simulink model "model_5LinkWalking_NODS"  (R2022b)
settings: Solver=VariableStepAuto  StartTime=0.0  StopTime=Tf  FixedStep=1e-5  MaxStep=1e-3  RelTol=1e-12  AbsTol=1e-8
values from neighbouring files (symbols this model uses):
  dq0 = [ocl_traj.simout(N,6); ocl_traj.simout(N,7); ocl_traj.simout(N,8); ocl_traj.simout(N,9); ocl_traj.simout(N,10)]    [run_walking_simulation.m]    (also in run_walking_simulation_parallel.m; search_delta_bar_parallel.m)
  gains = [K_p,K_d,K_p,K_d,K_p,K_d,K_p,K_d,K_p,K_d]    [main.m]
  init_flag = [-1; 0; ocl_traj.x_sw(1); init_t_mode_change; alpha_ref(1); 0; y_g_curr]    [run_walking_simulation.m]
  Initial_state = [q0;dq0]    [run_walking_simulation.m]    (also in run_walking_simulation_parallel.m; search_delta_bar_parallel.m)
  inputs_ref = [step_alpha_ref, step_inputs_ref]    [run_walking_simulation.m]
  joint_angles_ref = [ocl_traj.time, ocl_traj.simout, alpha_ref]    [run_walking_simulation.m]    (also in run_walking_simulation_parallel.m; search_delta_bar_parallel.m)
  landing_ref = [landing_traj.time, landing_traj.simout, alpha_ref_landing]    [run_walking_simulation.m]    (also in run_walking_simulation_parallel.m; search_delta_bar_parallel.m)
  param = [params.m1; params.m2; params.m5; params.l1; params.l2; params.l5; params.g; params.I1; params.I2; params.I5; params.r_k; params.r_h; params.k_ba; params.phi_h0; params.phi_k0]    [main.m]    (also in run_walking_simulation.m; run_walking_simulation_parallel.m)
  q0 = [ocl_traj.simout(N,1); ocl_traj.simout(N,2); ocl_traj.simout(N,3); ocl_traj.simout(N,4); ocl_traj.simout(N,5)]    [run_walking_simulation.m]    (also in run_walking_simulation_parallel.m; search_delta_bar_parallel.m)
  sample_time = 0.001    [run_walking_simulation.m]    (also in run_walking_simulation_parallel.m; search_delta_bar_parallel.m)
undefined symbols (not defined in the file or in its folder): uneven_terrain
libraries: simulink x2
(part 1 of 2)
settings Model: SimulationMode=accelerator  Creator=yamakita_lab  LastModifiedBy=mmpel
settings SolverCC: AutoScaleAbsTol=off  AlgebraicLoopSolver=TrustRegion
settings DataIOCC: ReturnWorkspaceOutputs=off
settings DebuggingCC: ParameterPrecisionLossMsg=none  UnconnectedInputMsg=warning  UnconnectedOutputMsg=warning  UnconnectedLineMsg=warning  SFMachineParentedDataDiag=warning  ArithmeticOperatorsInVariantConditions=warning
settings ModelReferenceCC: EnableRefExpFcnMdlSchedulingChecks=on
settings SFSimCC: SimUseLocalCustomCode=off  CustomCodeUndefinedFunction=UseInterfaceOnly
settings RTWCC: RTWUseLocalCustomCode=off  DLArmComputeVersion=19.05

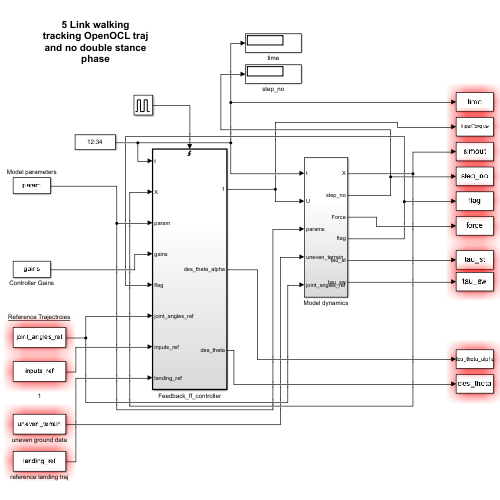
[thumbnail: Simulink's stored preview of the top-level diagram]
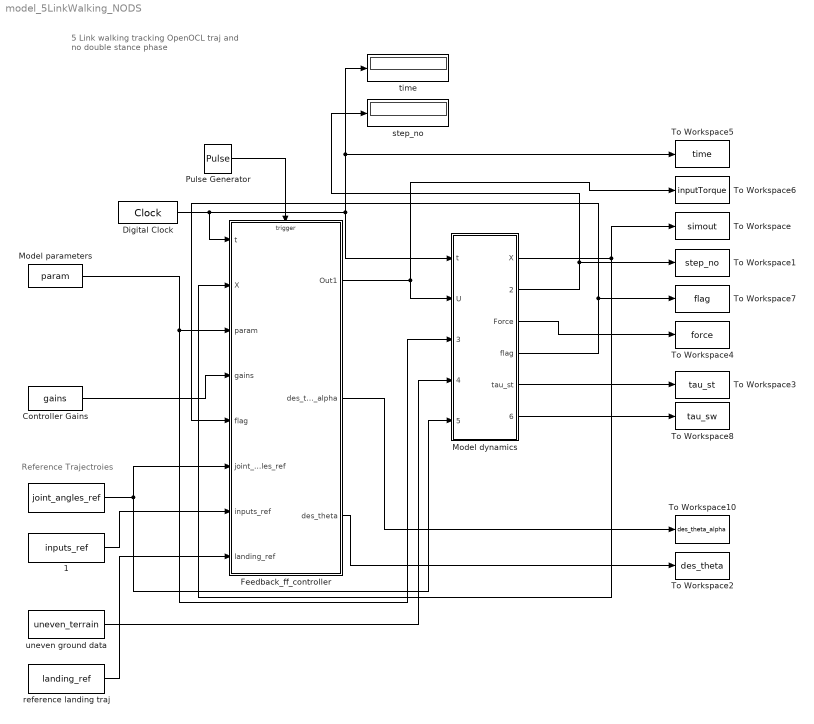
== system model_5LinkWalking_NODS ==
  note: Reference Trajectroies
  note: 5 Link walking tracking OpenOCL traj and no double stance phase
  " " : Constant  Value=joint_angles_ref
  " 1" : Constant  Value=inputs_ref
  Controller Gains : Constant  Value=gains
  Digital Clock : DigitalClock  SampleTime=1e-4
  Feedback_ff_controller : Subsystem  TreatAsAtomicUnit=on
  Model dynamics : Subsystem
  Model parameters : Constant  Value=param  OutDataTypeStr=double
  Pulse Generator : DiscretePulseGenerator  PulseType=Time based  Period=5e-4  PulseWidth=5
  To Workspace : ToWorkspace  VariableName=simout  SampleTime=sample_time
  To Workspace1 : ToWorkspace  VariableName=step_no  SampleTime=sample_time
  To Workspace10 : ToWorkspace  VariableName=des_theta_alpha  SampleTime=sample_time
  To Workspace2 : ToWorkspace  VariableName=des_theta  SampleTime=sample_time
  To Workspace3 : ToWorkspace  VariableName=tau_st  SampleTime=sample_time
  To Workspace4 : ToWorkspace  VariableName=force  SampleTime=sample_time
  To Workspace5 : ToWorkspace  VariableName=time  SampleTime=sample_time
  To Workspace6 : ToWorkspace  VariableName=inputTorque  SampleTime=sample_time
  To Workspace7 : ToWorkspace  VariableName=flag  SampleTime=sample_time
  To Workspace8 : ToWorkspace  VariableName=tau_sw  SampleTime=sample_time
  reference landing traj : Constant  Value=landing_ref
  step_no : Display
  time : Display
  uneven ground data : Constant  Value=uneven_terrain  OutDataTypeStr=Bus: uneven_terrain_bus
  wires:
  Feedback_ff_controller/1(Out1) -> Model dynamics/2(U), To Workspace6/1
  Model dynamics/1(X) -> To Workspace/1, Feedback_ff_controller/2(X)
  Digital Clock/1 -> time/1, To Workspace5/1, Model dynamics/1(t), Feedback_ff_controller/1(t)
  Model dynamics/2(step_no) -> step_no/1, To Workspace1/1
  Model dynamics/3(Force) -> To Workspace4/1
  Model parameters/1 -> Model dynamics/3(params), Feedback_ff_controller/3(param)
  Controller Gains/1 -> Feedback_ff_controller/4(gains)
  Model dynamics/4(flag) -> To Workspace7/1, Feedback_ff_controller/5(flag)
  " "/1 -> Model dynamics/5(joint_angles_ref), Feedback_ff_controller/6(joint_angles_ref)
  Pulse Generator/1 -> Feedback_ff_controller/Trigger
  Model dynamics/5(tau_st) -> To Workspace3/1
  Model dynamics/6(tau_sw) -> To Workspace8/1
  " 1"/1 -> Feedback_ff_controller/7(inputs_ref)
  Feedback_ff_controller/2(des_theta_alpha) -> To Workspace10/1
  Feedback_ff_controller/3(des_theta) -> To Workspace2/1
  uneven ground data/1 -> Model dynamics/4(uneven_terrain)
  reference landing traj/1 -> Feedback_ff_controller/8(landing_ref)

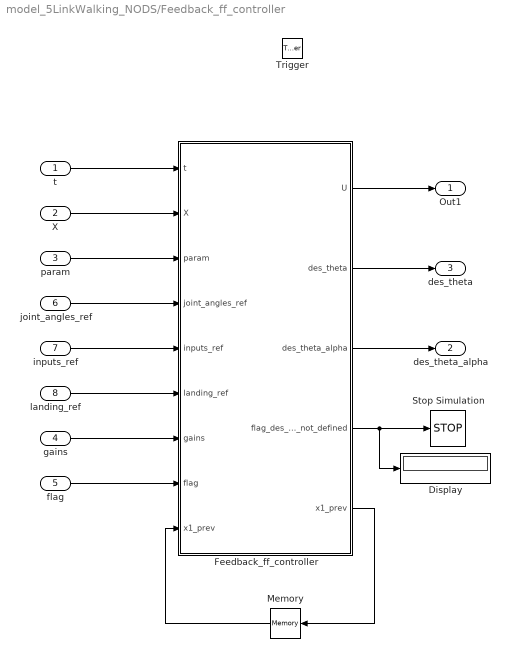
== system model_5LinkWalking_NODS/Feedback_ff_controller ==
  t : Inport
  X : Inport  Port=2
  param : Inport  Port=3
  gains : Inport  Port=4
  flag : Inport  Port=5
  joint_angles_ref : Inport  Port=6
  inputs_ref : Inport  Port=7
  landing_ref : Inport  Port=8
  Trigger : TriggerPort  VariantControl=Variant  PortDimensions=1
  Display : Display
  Feedback_ff_controller : MATLAB Function  TreatAsAtomicUnit=on
  Memory : Memory  InitialCondition=[0, 0]  InheritSampleTime=on
  Stop Simulation : Stop
  Out1 : Outport  VectorParamsAs1DForOutWhenUnconnected=off
  des_theta_alpha : Outport  Port=2  InitialOutput=[q0; dq0; 0]  VectorParamsAs1DForOutWhenUnconnected=off
  des_theta : Outport  Port=3  InitialOutput=[q0; dq0]  VectorParamsAs1DForOutWhenUnconnected=off
  wires:
  Feedback_ff_controller/1(U) -> Out1/1
  t/1 -> Feedback_ff_controller/1(t)
  X/1 -> Feedback_ff_controller/2(X)
  param/1 -> Feedback_ff_controller/3(param)
  Memory/1 -> Feedback_ff_controller/9("x1_prev ")
  Feedback_ff_controller/5(x1_prev) -> Memory/1
  gains/1 -> Feedback_ff_controller/7(gains)
  flag/1 -> Feedback_ff_controller/8(flag)
  joint_angles_ref/1 -> Feedback_ff_controller/4(joint_angles_ref)
  inputs_ref/1 -> Feedback_ff_controller/5(inputs_ref)
  Feedback_ff_controller/3(des_theta_alpha) -> des_theta_alpha/1
  Feedback_ff_controller/2(des_theta) -> des_theta/1
  landing_ref/1 -> Feedback_ff_controller/6(landing_ref)
  Feedback_ff_controller/4(flag_des_theta_not_defined) -> Display/1, Stop Simulation/1

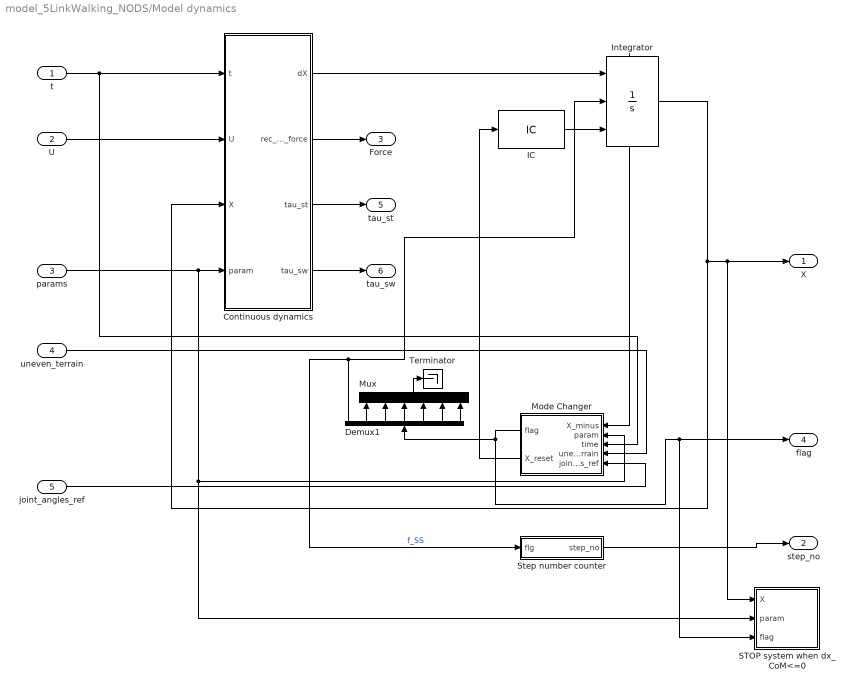
== system model_5LinkWalking_NODS/Model dynamics ==
  t : Inport
  U : Inport  Port=2
  params : Inport  Port=3
  uneven_terrain : Inport  Port=4
  joint_angles_ref : Inport  Port=5
  Continuous dynamics : MATLAB Function  TreatAsAtomicUnit=on
  Demux1 : Demux  Outputs=7
  IC : InitialCondition  Value=Initial_state
  Integrator : Integrator  ExternalReset=rising  InitialConditionSource=external  ShowStatePort=on
  Mode Changer : Subsystem
  Mux : Mux  Inputs=6
  STOP system when dx_CoM<=0 : Subsystem
  Step number counter : Subsystem
  Terminator : Terminator
  X : Outport  VectorParamsAs1DForOutWhenUnconnected=off
  step_no : Outport  Port=2  VectorParamsAs1DForOutWhenUnconnected=off
  Force : Outport  Port=3  VectorParamsAs1DForOutWhenUnconnected=off
  flag : Outport  Port=4
  tau_st : Outport  Port=5  VectorParamsAs1DForOutWhenUnconnected=off
  tau_sw : Outport  Port=6  VectorParamsAs1DForOutWhenUnconnected=off
  wires:
  IC/1 -> Integrator/3
  Integrator/State -> Mode Changer/1(X_minus)
  Continuous dynamics/1(dX) -> Integrator/1
  params/1 -> Continuous dynamics/4(param), STOP system when dx_CoM<=0/2(param), Mode Changer/2("param ")
  U/1 -> Continuous dynamics/2(U)
  t/1 -> Continuous dynamics/1(t), Mode Changer/3(time)
  Integrator/1 -> STOP system when dx_CoM<=0/1(X), X/1, Continuous dynamics/3(X)
  Mode Changer/2(X_reset) -> IC/1
  Mode Changer/1(flag) -> STOP system when dx_CoM<=0/3(flag), flag/1, Demux1/1
  Demux1/1 -> Integrator/2, Step number counter/1(flg)  "f_SS"
  Step number counter/1(step_no) -> step_no/1
  Continuous dynamics/2(rec_cs_force) -> Force/1
  Continuous dynamics/3(tau_st) -> tau_st/1
  Continuous dynamics/4(tau_sw) -> tau_sw/1
  Demux1/2 -> Mux/1
  Demux1/3 -> Mux/2
  Demux1/4 -> Mux/3
  Demux1/5 -> Mux/4
  Demux1/6 -> Mux/5
  Mux/1 -> Terminator/1
  uneven_terrain/1 -> Mode Changer/4(uneven_terrain)
  Demux1/7 -> Mux/6
  joint_angles_ref/1 -> Mode Changer/5(joint_angles_ref)

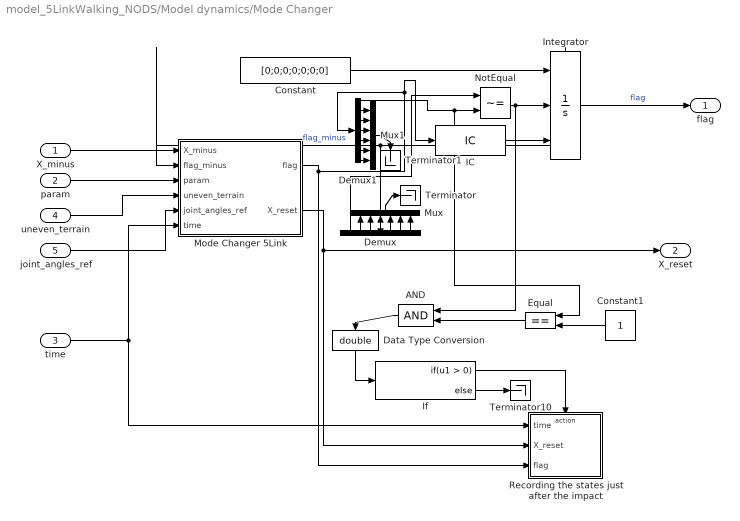
== system model_5LinkWalking_NODS/Model dynamics/Mode Changer ==
  X_minus : Inport
  "param " : Inport  Port=2
  time : Inport  Port=3
  uneven_terrain : Inport  Port=4
  joint_angles_ref : Inport  Port=5
  AND : Logic  IconShape=distinctive  AllPortsSameDT=off  OutDataTypeStr=boolean
  Constant : Constant  Value=[0;0;0;0;0;0;0]
  Constant1 : Constant
  Data Type Conversion : DataTypeConversion  OutDataTypeStr=double  SaturateOnIntegerOverflow=off  RndMeth=Floor
  Demux : Demux  Outputs=7
  Demux1 : Demux  Outputs=7
  Equal : RelationalOperator  Operator===  OutDataTypeStr=boolean  RndMeth=Simplest  InputSameDT=off
  IC : InitialCondition  Value=init_flag
  If : If
  Integrator : Integrator  ExternalReset=rising  InitialConditionSource=external  ShowStatePort=on
  Mode Changer 5Link : MATLAB Function  TreatAsAtomicUnit=on
  Mux : Mux  Inputs=6
  Mux1 : Mux  Inputs=6
  NotEqual : RelationalOperator  Operator=~=  OutDataTypeStr=boolean  RndMeth=Simplest  InputSameDT=off
  Recording the states just after the impact : Subsystem  TreatAsAtomicUnit=on
  Terminator : Terminator
  Terminator1 : Terminator
  Terminator10 : Terminator
  flag : Outport  VectorParamsAs1DForOutWhenUnconnected=off
  X_reset : Outport  Port=2  VectorParamsAs1DForOutWhenUnconnected=off
  wires:
  X_minus/1 -> Mode Changer 5Link/1(X_minus)
  IC/1 -> Integrator/3
  Integrator/State -> Mode Changer 5Link/2(flag_minus), Demux/1  "flag_minus"
  "param "/1 -> Mode Changer 5Link/3(param)
  Mode Changer 5Link/1(flag) -> Demux1/1, IC/1, Recording the states just after the impact/3(flag)
  Constant/1 -> Integrator/1
  NotEqual/1 -> AND/1, Integrator/2
  Integrator/1 -> flag/1  "flag"
  Mode Changer 5Link/2(X_reset) -> Recording the states just after the impact/2(X_reset), X_reset/1
  Demux/1 -> NotEqual/1
  time/1 -> Mode Changer 5Link/6(time), Recording the states just after the impact/1(time)
  Demux1/1 -> Equal/1, NotEqual/2
  If/1 -> Recording the states just after the impact/Action
  If/2 -> Terminator10/1
  Data Type Conversion/1 -> If/1
  AND/1 -> Data Type Conversion/1
  Equal/1 -> AND/2
  Constant1/1 -> Equal/2
  uneven_terrain/1 -> Mode Changer 5Link/4(uneven_terrain)
  Demux/2 -> Mux/1
  Demux/3 -> Mux/2
  Demux/4 -> Mux/3
  Demux/5 -> Mux/4
  Demux/6 -> Mux/5
  Demux/7 -> Mux/6
  Mux/1 -> Terminator/1
  Demux1/2 -> Mux1/1
  Demux1/3 -> Mux1/2
  Demux1/4 -> Mux1/3
  Demux1/5 -> Mux1/4
  Demux1/6 -> Mux1/5
  Demux1/7 -> Mux1/6
  Mux1/1 -> Terminator1/1
  joint_angles_ref/1 -> Mode Changer 5Link/5(joint_angles_ref)

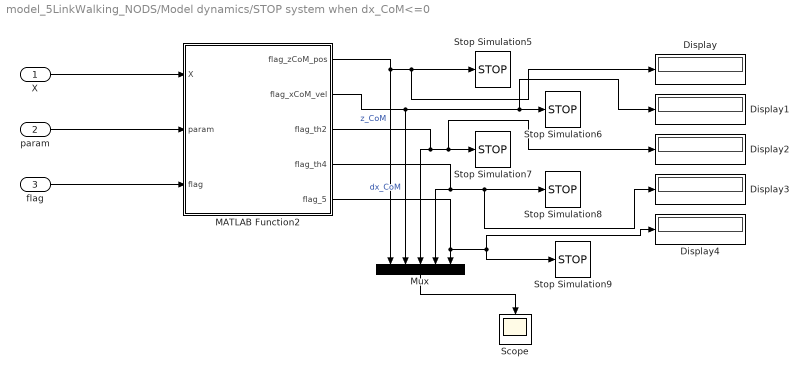
== system model_5LinkWalking_NODS/Model dynamics/STOP system when dx_CoM<=0 ==
  X : Inport
  param : Inport  Port=2
  flag : Inport  Port=3
  Display{,1..4} (5 alike) : Display
  MATLAB Function2 : MATLAB Function  TreatAsAtomicUnit=on
  Mux : Mux  Inputs=5
  Scope : Scope
  Stop Simulation{5..9} (5 alike) : Stop
  wires:
  X/1 -> MATLAB Function2/1(X)
  param/1 -> MATLAB Function2/2(param)
  flag/1 -> MATLAB Function2/3(flag)
  MATLAB Function2/1(flag_zCoM_pos) -> Mux/1, Display/1, Stop Simulation5/1  "z_CoM"
  MATLAB Function2/2(flag_xCoM_vel) -> Display1/1, Stop Simulation6/1, Mux/2  "dx_CoM"
  MATLAB Function2/4(flag_th4) -> Mux/4, Display3/1, Stop Simulation8/1
  Mux/1 -> Scope/1
  MATLAB Function2/3(flag_th2) -> Display2/1, Stop Simulation7/1, Mux/3
  MATLAB Function2/5(flag_5) -> Display4/1, Stop Simulation9/1, Mux/5

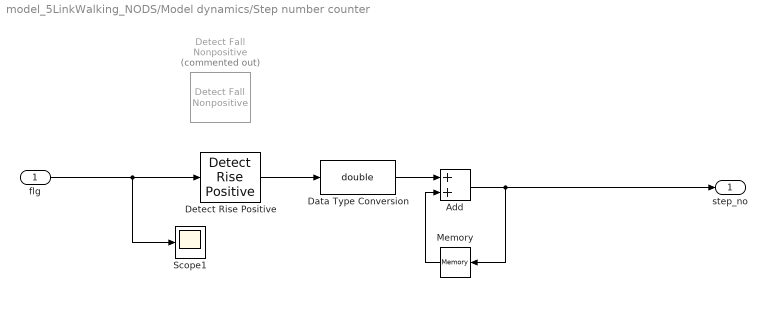
== system model_5LinkWalking_NODS/Model dynamics/Step number counter ==
  flg : Inport  SampleTime=sample_time
  Add : Sum
  Data Type Conversion : DataTypeConversion  OutDataTypeStr=double  SaturateOnIntegerOverflow=off  RndMeth=Floor
  Detect Fall Nonpositive : simulink/Logic and Bit Operations/Detect Fall Nonpositive  Commented=on  vinit=1  OutDataTypeStr=boolean
  Detect Rise Positive : simulink/Logic and Bit Operations/Detect Rise Positive  vinit=-1  OutDataTypeStr=boolean
  Memory : Memory  InheritSampleTime=on
  Scope1 : Scope
  step_no : Outport  VectorParamsAs1DForOutWhenUnconnected=off
  wires:
  Add/1 -> step_no/1, Memory/1
  Memory/1 -> Add/2
  flg/1 -> Detect Rise Positive/1, Scope1/1
  Data Type Conversion/1 -> Add/1
  Detect Rise Positive/1 -> Data Type Conversion/1

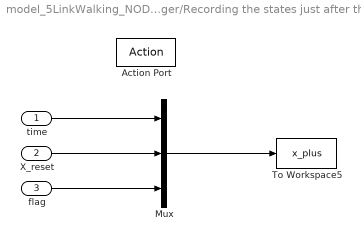
== system model_5LinkWalking_NODS/Model dynamics/Mode Changer/Recording the states just after the impact ==
  time : Inport
  X_reset : Inport  Port=2
  flag : Inport  Port=3
  Action Port : ActionPort  ActionPortLabel=if(u1 > 0)
  Mux : Mux  Inputs=3
  To Workspace5 : ToWorkspace  VariableName=x_plus  SampleTime=-1
  wires:
  time/1 -> Mux/1
  X_reset/1 -> Mux/2
  flag/1 -> Mux/3
  Mux/1 -> To Workspace5/1

== matlab function model_5LinkWalking_NODS/Model dynamics/Continuous dynamics ==
  data: t input; U input; dX output; rec_cs_force output; X input; param input; tau_st output; tau_sw output
function [dX, rec_cs_force, tau_st, tau_sw] = fcn(t, U, X, param)

%% variables
th1 = X(1);
th2 = X(2);
th3 = X(3);
th4 = X(4);
th5 = X(5);

dth1 = X(6);
dth2 = X(7);
dth3 = X(8);
dth4 = X(9);
dth5 = X(10);

q = [th1;th2;th3;th4;th5];
dq = [dth1;dth2;dth3;dth4;dth5];

%% parameters

m1 = param(1);
m2 = param(2);
m3 = m2;
m4 = m1;
m5 = param(3);

l1 = param(4);
l2 = param(5);
l5 = param(6);
l3 = l2;
l4 = l1;

gravi = param(7);
I1 = param(8);
I2 = param(9);
I5 = param(10);
I3 = I1;
I4 = I2;

r_k = param(11);
r_h = param(12);
k_ba = param(13);
phi_h0 = param(14);
phi_k0 = param(15);

%% flags
% f_SS = flag(1); % indicates which stance phase it is
% foot = flag(2); % location of the stance foot
% foot_prev = flag(3); % previous location of the stance foot

%% Inertia Matrix
MM = MM_matrix(X,param);

%% Centrifugal force · Coriolis force Vector
CC = zeros(5,1);

CC(1, 1) = - (dth2^2*l1*l3*m3*sin(th2 + th3))/2 - dth2^2*l1*l3*m4*sin(th2 + th3) - (dth3^2*l1*l3*m3*sin(th2 + th3))/2 - dth3^2*l1*l3*m4*sin(th2 + th3) - (dth2^2*l1*l5*m5*sin(th2 + th5))/2 - (dth3^2*l2*l4*m4*sin(th3 + th4))/2 - (dth4^2*l2*l4*m4*sin(th3 + th4))/2 - (dth5^2*l1*l5*m5*sin(th2 + th5))/2 - (dth2^2*l1*l2*m2*sin(th2))/2 - dth2^2*l1*l2*m3*sin(th2) - dth2^2*l1*l2*m4*sin(th2) - dth2^2*l1*l2*m5*sin(th2) - (dth3^2*l2*l3*m3*sin(th3))/2 - dth3^2*l2*l3*m4*sin(th3) - (dth4^2*l3*l4*m4*sin(th4))/2 - (dth5^2*l2*l5*m5*sin(th5))/2 - (dth2^2*l1*l4*m4*sin(th2 + th3 + th4))/2 - (dth3^2*l1*l4*m4*sin(th2 + th3 + th4))/2 - (dth4^2*l1*l4*m4*sin(th2 + th3 + th4))/2 - dth1*dth2*l1*l3*m3*sin(th2 + th3) - 2*dth1*dth2*l1*l3*m4*sin(th2 + th3) - dth1*dth3*l1*l3*m3*sin(th2 + th3) - 2*dth1*dth3*l1*l3*m4*sin(th2 + th3) - dth2*dth3*l1*l3*m3*sin(th2 + th3) - 2*dth2*dth3*l1*l3*m4*sin(th2 + th3) - dth1*dth2*l1*l5*m5*sin(th2 + th5) - dth1*dth3*l2*l4*m4*sin(th3 + th4) - dth1*dth4*l2*l4*m4*sin(th3 + th4) - dth2*dth3*l2*l4*m4*sin(th3 + th4) - dth2*dth4*l2*l4*m4*sin(th3 + th4) - dth1*dth5*l1*l5*m5*sin(th2 + th5) - dth3*dth4*l2*l4*m4*sin(th3 + th4) - dth2*dth5*l1*l5*m5*sin(th2 + th5) - dth1*dth2*l1*l2*m2*sin(th2) - 2*dth1*dth2*l1*l2*m3*sin(th2) - 2*dth1*dth2*l1*l2*m4*sin(th2) - 2*dth1*dth2*l1*l2*m5*sin(th2) - dth1*dth3*l2*l3*m3*sin(th3) - 2*dth1*dth3*l2*l3*m4*sin(th3) - dth2*dth3*l2*l3*m3*sin(th3) - 2*dth2*dth3*l2*l3*m4*sin(th3) - dth1*dth4*l3*l4*m4*sin(th4) - dth2*dth4*l3*l4*m4*sin(th4) - dth3*dth4*l3*l4*m4*sin(th4) - dth1*dth5*l2*l5*m5*sin(th5) - dth2*dth5*l2*l5*m5*sin(th5) - dth1*dth2*l1*l4*m4*sin(th2 + th3 + th4) - dth1*dth3*l1*l4*m4*sin(th2 + th3 + th4) - dth1*dth4*l1*l4*m4*sin(th2 + th3 + th4) - dth2*dth3*l1*l4*m4*sin(th2 + th3 + th4) - dth2*dth4*l1*l4*m4*sin(th2 + th3 + th4) - dth3*dth4*l1*l4*m4*sin(th2 + th3 + th4);
CC(2, 1) = (dth1^2*l1*l3*m3*sin(th2 + th3))/2 + dth1^2*l1*l3*m4*sin(th2 + th3) + (dth1^2*l1*l5*m5*sin(th2 + th5))/2 - (dth3^2*l2*l4*m4*sin(th3 + th4))/2 - (dth4^2*l2*l4*m4*sin(th3 + th4))/2 + (dth1^2*l1*l2*m2*sin(th2))/2 + dth1^2*l1*l2*m3*sin(th2) + dth1^2*l1*l2*m4*sin(th2) + dth1^2*l1*l2*m5*sin(th2) - (dth3^2*l2*l3*m3*sin(th3))/2 - dth3^2*l2*l3*m4*sin(th3) - (dth4^2*l3*l4*m4*sin(th4))/2 - (dth5^2*l2*l5*m5*sin(th5))/2 + (dth1^2*l1*l4*m4*sin(th2 + th3 + th4))/2 - dth1*dth3*l2*l4*m4*sin(th3 + th4) - dth1*dth4*l2*l4*m4*sin(th3 + th4) - dth2*dth3*l2*l4*m4*sin(th3 + th4) - dth2*dth4*l2*l4*m4*sin(th3 + th4) - dth3*dth4*l2*l4*m4*sin(th3 + th4) - dth1*dth3*l2*l3*m3*sin(th3) - 2*dth1*dth3*l2*l3*m4*sin(th3) - dth2*dth3*l2*l3*m3*sin(th3) - 2*dth2*dth3*l2*l3*m4*sin(th3) - dth1*dth4*l3*l4*m4*sin(th4) - dth2*dth4*l3*l4*m4*sin(th4) - dth3*dth4*l3*l4*m4*sin(th4) - dth1*dth5*l2*l5*m5*sin(th5) - dth2*dth5*l2*l5*m5*sin(th5);
CC(3, 1) = (dth1^2*l1*l3*m3*sin(th2 + th3))/2 + dth1^2*l1*l3*m4*sin(th2 + th3) + (dth1^2*l2*l4*m4*sin(th3 + th4))/2 + (dth2^2*l2*l4*m4*sin(th3 + th4))/2 + (dth1^2*l2*l3*m3*sin(th3))/2 + dth1^2*l2*l3*m4*sin(th3) + (dth2^2*l2*l3*m3*sin(th3))/2 + dth2^2*l2*l3*m4*sin(th3) - (dth4^2*l3*l4*m4*sin(th4))/2 + (dth1^2*l1*l4*m4*sin(th2 + th3 + th4))/2 + dth1*dth2*l2*l4*m4*sin(th3 + th4) + dth1*dth2*l2*l3*m3*sin(th3) + 2*dth1*dth2*l2*l3*m4*sin(th3) - dth1*dth4*l3*l4*m4*sin(th4) - dth2*dth4*l3*l4*m4*sin(th4) - dth3*dth4*l3*l4*m4*sin(th4);
CC(4, 1) = (l4*m4*(dth1^2*l2*sin(th3 + th4) + dth2^2*l2*sin(th3 + th4) + dth1^2*l3*sin(th4) + dth2^2*l3*sin(th4) + dth3^2*l3*sin(th4) + dth1^2*l1*sin(th2 + th3 + th4) + 2*dth1*dth2*l2*sin(th3 + th4) + 2*dth1*dth2*l3*sin(th4) + 2*dth1*dth3*l3*sin(th4) + 2*dth2*dth3*l3*sin(th4)))/2;
CC(5, 1) = (l5*m5*(dth1^2*l1*sin(th2 + th5) + dth1^2*l2*sin(th5) + dth2^2*l2*sin(th5) + 2*dth1*dth2*l2*sin(th5)))/2;

%% Gravity Vector
GG = zeros(5,1);

GG(1, 1) = (m3*(l2*cos(th1 + th2) + l1*cos(th1) + (l3*cos(th1 + th2 + th3))/2) + m5*(l2*cos(th1 + th2) + l1*cos(th1) + (l5*cos(th1 + th2 + th5))/2) + m2*((l2*cos(th1 + th2))/2 + l1*cos(th1)) + m4*((l4*cos(th1 + th2 + th3 + th4))/2 + l2*cos(th1 + th2) + l1*cos(th1) + l3*cos(th1 + th2 + th3)) + (l1*m1*cos(th1))/2)*gravi;
GG(2, 1) = (m3*(l2*cos(th1 + th2) + (l3*cos(th1 + th2 + th3))/2) + m5*(l2*cos(th1 + th2) + (l5*cos(th1 + th2 + th5))/2) + m4*((l4*cos(th1 + th2 + th3 + th4))/2 + l2*cos(th1 + th2) + l3*cos(th1 + th2 + th3)) + (l2*m2*cos(th1 + th2))/2)*gravi;
GG(3, 1) = (m4*((l4*cos(th1 + th2 + th3 + th4))/2 + l3*cos(th1 + th2 + th3)) + (l3*m3*cos(th1 + th2 + th3))/2)*gravi;
GG(4, 1) = ((l4*m4*cos(th1 + th2 + th3 + th4))/2)*gravi;
GG(5, 1) = ((l5*m5*cos(th1 + th2 + th5))/2)*gravi;

%% input torques mapping matrix
S = [
    1,0,0,0,0;
    0,1,0,0,0;
    0,0,1,0,0;
    0,0,0,1,0;
    0,0,-1,0,1;];

%% Biarticular Spring Force

% Calculating the knee and hip angles
% We meed wrapTo2Pi() because some angles increase to inf due to the reset
% function eg. th1 and th5

phi_h_st = mod(th5 - pi, 2*pi); % angle between torso and stance thigh
phi_k_st = mod(pi - th2, 2*pi); % angle between stance thigh and shank
phi_h_sw = mod(th5 - th3, 2*pi); % angle between torso and swing thigh
phi_k_sw = mod(th4 - pi, 2*pi); % angle between swing thigh and shank

% Calculating the elongation in the springs
delta_l_st = r_h*(phi_h_st - phi_h0) - r_k*(phi_k_st - phi_k0); % elongation of BA in stance leg [m]
delta_l_sw = r_h*(phi_h_sw - phi_h0) - r_k*(phi_k_sw - phi_k0); % elongation of BA in swing leg [m]

% torques due to BA in stance leg
tau_st = [
    0;
    -k_ba*delta_l_st*r_k;
    0;
    0;
    -k_ba*delta_l_st*r_h];

% torques due to BA in swing leg
tau_sw = [
    0;
    0;
    k_ba*delta_l_sw*r_h;
    k_ba*delta_l_sw*r_k;
    -k_ba*delta_l_sw*r_h];

springForce = tau_st + tau_sw;
%% Constraint Force Calculation (in case of Double Stance)
J_c = zeros(2,5);
J_c(1,1) = - l4*sin(th1 + th2 + th3 + th4) - l3*sin(th1 + th2 + th3) - l2*sin(th1 + th2) - l1*sin(th1);
J_c(1,2) = - l4*sin(th1 + th2 + th3 + th4) - l3*sin(th1 + th2 + th3) - l2*sin(th1 + th2);
J_c(1,3) = - l4*sin(th1 + th2 + th3 + th4) - l3*sin(th1 + th2 + th3);
J_c(1,4) = - l4*sin(th1 + th2 + th3 + th4);
J_c(1,5) = 0;

J_c(2,1) = l4*cos(th1 + th2 + th3 + th4) + l2*cos(th1 + th2) + l1*cos(th1) + l3*cos(th1 + th2 + th3);
J_c(2,2) = l4*cos(th1 + th2 + th3 + th4) + l2*cos(th1 + th2) + l3*cos(th1 + th2 + th3);
J_c(2,3) = l4*cos(th1 + th2 + th3 + th4) + l3*cos(th1 + th2 + th3);
J_c(2,4) = l4*cos(th1 + th2 + th3 + th4);
J_c(2,5) = 0;

dJ_c = zeros(2,5);
dJ_c(1,1) = - dth3*(l4*cos(th1 + th2 + th3 + th4) + l3*cos(th1 + th2 + th3)) - dth1*(l4*cos(th1 + th2 + th3 + th4) + l2*cos(th1 + th2) + l1*cos(th1) + l3*cos(th1 + th2 + th3)) - dth2*(l4*cos(th1 + th2 + th3 + th4) + l2*cos(th1 + th2) + l3*cos(th1 + th2 + th3)) - dth4*l4*cos(th1 + th2 + th3 + th4);
dJ_c(1,2) = - dth3*(l4*cos(th1 + th2 + th3 + th4) + l3*cos(th1 + th2 + th3)) - dth1*(l4*cos(th1 + th2 + th3 + th4) + l2*cos(th1 + th2) + l3*cos(th1 + th2 + th3)) - dth2*(l4*cos(th1 + th2 + th3 + th4) + l2*cos(th1 + th2) + l3*cos(th1 + th2 + th3)) - dth4*l4*cos(th1 + th2 + th3 + th4);
dJ_c(1,3) = - dth1*(l4*cos(th1 + th2 + th3 + th4) + l3*cos(th1 + th2 + th3)) - dth2*(l4*cos(th1 + th2 + th3 + th4) + l3*cos(th1 + th2 + th3)) - dth3*(l4*cos(th1 + th2 + th3 + th4) + l3*cos(th1 + th2 + th3)) - dth4*l4*cos(th1 + th2 + th3 + th4);
dJ_c(1,4) = - l4*cos(th1 + th2 + th3 + th4)*(dth1 + dth2 + dth3 + dth4);
dJ_c(1,5) = 0;

dJ_c(2,1) = - dth2*(l4*sin(th1 + th2 + th3 + th4) + l2*sin(th1 + th2) + l3*sin(th1 + th2 + th3)) - dth3*(l4*sin(th1 + th2 + th3 + th4) + l3*sin(th1 + th2 + th3)) - dth1*(l4*sin(th1 + th2 + th3 + th4) + l2*sin(th1 + th2) + l1*sin(th1) + l3*sin(th1 + th2 + th3)) - dth4*l4*sin(th1 + th2 + th3 + th4);
dJ_c(2,2) = - dth1*(l4*sin(th1 + th2 + th3 + th4) + l2*sin(th1 + th2) + l3*sin(th1 + th2 + th3)) - dth2*(l4*sin(th1 + th2 + th3 + th4) + l2*sin(th1 + th2) + l3*sin(th1 + th2 + th3)) - dth3*(l4*sin(th1 + th2 + th3 + th4) + l3*sin(th1 + th2 + th3)) - dth4*l4*sin(th1 + th2 + th3 + th4);
dJ_c(2,3) = - dth1*(l4*sin(th1 + th2 + th3 + th4) + l3*sin(th1 + th2 + th3)) - dth2*(l4*sin(th1 + th2 + th3 + th4) + l3*sin(th1 + th2 + th3)) - dth3*(l4*sin(th1 + th2 + th3 + th4) + l3*sin(th1 + th2 + th3)) - dth4*l4*sin(th1 + th2 + th3 + th4);
dJ_c(2,4) = - l4*sin(th1 + th2 + th3 + th4)*(dth1 + dth2 + dth3 + dth4);
dJ_c(2,5) = 0;

constraint_force = zeros(2,1);
constraint_force = -inv(J_c*inv(MM)*J_c')*(J_c*inv(MM)*(S*U+tau_st+tau_sw-CC-GG)+dJ_c*dq);

%% Acceleration Calculation
% ddq = zeros(5,1);
% rec_cs_force = [0;0;0;0];

% switch_time = flag(4); % time when double stance phase begins
% if (f_SS == -1 && constraint_force(2) >= 0) || (f_SS == -1 && t - switch_time < 0.05) % second part is because right after impact, there might be some fluctuations so it disregards them for 0.01 secs
% % if f_SS == 0
%     ddq = inv(MM)*(- CC - GG + S*U + tau_sw + tau_st + transpose(J_c)*constraint_force);  
%     rec_cs_force = [constraint_force; 0;0];
% else
%     rec_cs_force = [0; 0; constraint_force];
%     constraint_force = [0; 0]; % don't constraint the swing foot if force in horizontal direction is pulling if its not right after the impact
%     ddq = inv(MM)*(- CC - GG + S*U + tau_st + tau_sw);
% end

rec_cs_force = [0; 0; constraint_force];
constraint_force = [0; 0]; % don't constraint the swing foot if force in horizontal direction is pulling if its not right after the impact
ddq = inv(MM)*(- CC - GG + S*U + tau_st + tau_sw);

%% Acceleration of CoM to visualize tracking of desired CoM acc.
% ddth1 = ddq(1);
% ddth2 = ddq(2);
% ddth3 = ddq(3);
% ddth4 = ddq(4);
% ddth5 = ddq(5);
% 
% x1 = foot;
% xG = (m4*(x1 + (l4*cos(th1 + th2 + th3 + th4))/2 + l2*cos(th1 + th2) + l1*cos(th1) + l3*cos(th1 + th2 + th3)) + m1*(x1 + (l1*cos(th1))/2) + m3*(x1 + l2*cos(th1 + th2) + l1*cos(th1) + (l3*cos(th1 + th2 + th3))/2) + m5*(x1 + l2*cos(th1 + th2) + l1*cos(th1) + (l5*cos(th1 + th2 + th5))/2) + m2*(x1 + (l1*cos(th1 + th2))/2 + l1*cos(th1)))/(m1 + m2 + m3 + m4 + m5);
% zG = (m3*(l2*sin(th1 + th2) + l1*sin(th1) + (l3*sin(th1 + th2 + th3))/2) + m5*(l2*sin(th1 + th2) + l1*sin(th1) + (l5*sin(th1 + th2 + th5))/2) + m2*((l2*sin(th1 + th2))/2 + l1*sin(th1)) + m4*((l4*sin(th1 + th2 + th3 + th4))/2 + l2*sin(th1 + th2) + l1*sin(th1) + l3*sin(th1 + th2 + th3)) + (l1*m1*sin(th1))/2)/(m1 + m2 + m3 + m4 + m5);
% 
% dxG = - (dth3*(m4*((l4*sin(th1 + th2 + th3 + th4))/2 + l3*sin(th1 + th2 + th3)) + (l3*m3*sin(th1 + th2 + th3))/2))/(m1 + m2 + m3 + m4 + m5) - (dth1*(m3*(l2*sin(th1 + th2) + l1*sin(th1) + (l3*sin(th1 + th2 + th3))/2) + m5*(l2*sin(th1 + th2) + l1*sin(th1) + (l5*sin(th1 + th2 + th5))/2) + m2*((l1*sin(th1 + th2))/2 + l1*sin(th1)) + m4*((l4*sin(th1 + th2 + th3 + th4))/2 + l2*sin(th1 + th2) + l1*sin(th1) + l3*sin(th1 + th2 + th3)) + (l1*m1*sin(th1))/2))/(m1 + m2 + m3 + m4 + m5) - (dth2*(m4*((l4*sin(th1 + th2 + th3 + th4))/2 + l2*sin(th1 + th2) + l3*sin(th1 + th2 + th3)) + m3*(l2*sin(th1 + th2) + (l3*sin(th1 + th2 + th3))/2) + m5*(l2*sin(th1 + th2) + (l5*sin(th1 + th2 + th5))/2) + (l1*m2*sin(th1 + th2))/2))/(m1 + m2 + m3 + m4 + m5) - (dth4*l4*m4*sin(th1 + th2 + th3 + th4))/(2*(m1 + m2 + m3 + m4 + m5)) - (dth5*l5*m5*sin(th1 + th2 + th5))/(2*(m1 + m2 + m3 + m4 + m5));
% dzG = (dth1*(m3*(l2*cos(th1 + th2) + l1*cos(th1) + (l3*cos(th1 + th2 + th3))/2) + m5*(l2*cos(th1 + th2) + l1*cos(th1) + (l5*cos(th1 + th2 + th5))/2) + m2*((l2*cos(th1 + th2))/2 + l1*cos(th1)) + m4*((l4*cos(th1 + th2 + th3 + th4))/2 + l2*cos(th1 + th2) + l1*cos(th1) + l3*cos(th1 + th2 + th3)) + (l1*m1*cos(th1))/2))/(m1 + m2 + m3 + m4 + m5) + (dth3*(m4*((l4*cos(th1 + th2 + th3 + th4))/2 + l3*cos(th1 + th2 + th3)) + (l3*m3*cos(th1 + th2 + th3))/2))/(m1 + m2 + m3 + m4 + m5) + (dth2*(m3*(l2*cos(th1 + th2) + (l3*cos(th1 + th2 + th3))/2) + m5*(l2*cos(th1 + th2) + (l5*cos(th1 + th2 + th5))/2) + m4*((l4*cos(th1 + th2 + th3 + th4))/2 + l2*cos(th1 + th2) + l3*cos(th1 + th2 + th3)) + (l2*m2*cos(th1 + th2))/2))/(m1 + m2 + m3 + m4 + m5) + (dth4*l4*m4*cos(th1 + th2 + th3 + th4))/(2*(m1 + m2 + m3 + m4 + m5)) + (dth5*l5*m5*cos(th1 + th2 + th5))/(2*(m1 + m2 + m3 + m4 + m5));
% 
% ddxG = - dth4*((dth1*l4*m4*cos(th1 + th2 + th3 + th4))/(2*(m1 + m2 + m3 + m4 + m5)) + (dth2*l4*m4*cos(th1 + th2 + th3 + th4))/(2*(m1 + m2 + m3 + m4 + m5)) + (dth3*l4*m4*cos(th1 + th2 + th3 + th4))/(2*(m1 + m2 + m3 + m4 + m5)) + (dth4*l4*m4*cos(th1 + th2 + th3 + th4))/(2*(m1 + m2 + m3 + m4 + m5))) - dth2*((dth3*(m4*((l4*cos(th1 + th2 + th3 + th4))/2 + l3*cos(th1 + th2 + th3)) + (l3*m3*cos(th1 + th2 + th3))/2))/(m1 + m2 + m3 + m4 + m5) + (dth1*(m3*(l2*cos(th1 + th2) + (l3*cos(th1 + th2 + th3))/2) + m5*(l2*cos(th1 + th2) + (l5*cos(th1 + th2 + th5))/2) + m4*((l4*cos(th1 + th2 + th3 + th4))/2 + l2*cos(th1 + th2) + l3*cos(th1 + th2 + th3)) + (l1*m2*cos(th1 + th2))/2))/(m1 + m2 + m3 + m4 + m5) + (dth2*(m3*(l2*cos(th1 + th2) + (l3*cos(th1 + th2 + th3))/2) + m5*(l2*cos(th1 + th2) + (l5*cos(th1 + th2 + th5))/2) + m4*((l4*cos(th1 + th2 + th3 + th4))/2 + l2*cos(th1 + th2) + l3*cos(th1 + th2 + th3)) + (l1*m2*cos(th1 + th2))/2))/(m1 + m2 + m3 + m4 + m5) + (dth4*l4*m4*cos(th1 + th2 + th3 + th4))/(2*(m1 + m2 + m3 + m4 + m5)) + (dth5*l5*m5*cos(th1 + th2 + th5))/(2*(m1 + m2 + m3 + m4 + m5))) - dth3*((dth1*(m4*((l4*cos(th1 + th2 + th3 + th4))/2 + l3*cos(th1 + th2 + th3)) + (l3*m3*cos(th1 + th2 + th3))/2))/(m1 + m2 + m3 + m4 + m5) + (dth2*(m4*((l4*cos(th1 + th2 + th3 + th4))/2 + l3*cos(th1 + th2 + th3)) + (l3*m3*cos(th1 + th2 + th3))/2))/(m1 + m2 + m3 + m4 + m5) + (dth3*(m4*((l4*cos(th1 + th2 + th3 + th4))/2 + l3*cos(th1 + th2 + th3)) + (l3*m3*cos(th1 + th2 + th3))/2))/(m1 + m2 + m3 + m4 + m5) + (dth4*l4*m4*cos(th1 + th2 + th3 + th4))/(2*(m1 + m2 + m3 + m4 + m5))) - dth1*((dth1*(m3*(l2*cos(th1 + th2) + l1*cos(th1) + (l3*cos(th1 + th2 + th3))/2) + m5*(l2*cos(th1 + th2) + l1*cos(th1) + (l5*cos(th1 + th2 + th5))/2) + m2*((l1*cos(th1 + th2))/2 + l1*cos(th1)) + m4*((l4*cos(th1 + th2 + th3 + th4))/2 + l2*cos(th1 + th2) + l1*cos(th1) + l3*cos(th1 + th2 + th3)) + (l1*m1*cos(th1))/2))/(m1 + m2 + m3 + m4 + m5) + (dth3*(m4*((l4*cos(th1 + th2 + th3 + th4))/2 + l3*cos(th1 + th2 + th3)) + (l3*m3*cos(th1 + th2 + th3))/2))/(m1 + m2 + m3 + m4 + m5) + (dth2*(m3*(l2*cos(th1 + th2) + (l3*cos(th1 + th2 + th3))/2) + m5*(l2*cos(th1 + th2) + (l5*cos(th1 + th2 + th5))/2) + m4*((l4*cos(th1 + th2 + th3 + th4))/2 + l2*cos(th1 + th2) + l3*cos(th1 + th2 + th3)) + (l1*m2*cos(th1 + th2))/2))/(m1 + m2 + m3 + m4 + m5) + (dth4*l4*m4*cos(th1 + th2 + th3 + th4))/(2*(m1 + m2 + m3 + m4 + m5)) + (dth5*l5*m5*cos(th1 + th2 + th5))/(2*(m1 + m2 + m3 + m4 + m5))) - dth5*((dth1*l5*m5*cos(th1 + th2 + th5))/(2*(m1 + m2 + m3 + m4 + m5)) + (dth2*l5*m5*cos(th1 + th2 + th5))/(2*(m1 + m2 + m3 + m4 + m5)) + (dth5*l5*m5*cos(th1 + th2 + th5))/(2*(m1 + m2 + m3 + m4 + m5))) - (ddth3*(m4*((l4*sin(th1 + th2 + th3 + th4))/2 + l3*sin(th1 + th2 + th3)) + (l3*m3*sin(th1 + th2 + th3))/2))/(m1 + m2 + m3 + m4 + m5) - (ddth1*(m3*(l2*sin(th1 + th2) + l1*sin(th1) + (l3*sin(th1 + th2 + th3))/2) + m5*(l2*sin(th1 + th2) + l1*sin(th1) + (l5*sin(th1 + th2 + th5))/2) + m2*((l1*sin(th1 + th2))/2 + l1*sin(th1)) + m4*((l4*sin(th1 + th2 + th3 + th4))/2 + l2*sin(th1 + th2) + l1*sin(th1) + l3*sin(th1 + th2 + th3)) + (l1*m1*sin(th1))/2))/(m1 + m2 + m3 + m4 + m5) - (ddth2*(m4*((l4*sin(th1 + th2 + th3 + th4))/2 + l2*sin(th1 + th2) + l3*sin(th1 + th2 + th3)) + m3*(l2*sin(th1 + th2) + (l3*sin(th1 + th2 + th3))/2) + m5*(l2*sin(th1 + th2) + (l5*sin(th1 + th2 + th5))/2) + (l1*m2*sin(th1 + th2))/2))/(m1 + m2 + m3 + m4 + m5) - (ddth4*l4*m4*sin(th1 + th2 + th3 + th4))/(2*(m1 + m2 + m3 + m4 + m5)) - (ddth5*l5*m5*sin(th1 + th2 + th5))/(2*(m1 + m2 + m3 + m4 + m5));
% ddzG = (ddth1*(m3*(l2*cos(th1 + th2) + l1*cos(th1) + (l3*cos(th1 + th2 + th3))/2) + m5*(l2*cos(th1 + th2) + l1*cos(th1) + (l5*cos(th1 + th2 + th5))/2) + m2*((l2*cos(th1 + th2))/2 + l1*cos(th1)) + m4*((l4*cos(th1 + th2 + th3 + th4))/2 + l2*cos(th1 + th2) + l1*cos(th1) + l3*cos(th1 + th2 + th3)) + (l1*m1*cos(th1))/2))/(m1 + m2 + m3 + m4 + m5) - dth3*((dth1*(m4*((l4*sin(th1 + th2 + th3 + th4))/2 + l3*sin(th1 + th2 + th3)) + (l3*m3*sin(th1 + th2 + th3))/2))/(m1 + m2 + m3 + m4 + m5) + (dth2*(m4*((l4*sin(th1 + th2 + th3 + th4))/2 + l3*sin(th1 + th2 + th3)) + (l3*m3*sin(th1 + th2 + th3))/2))/(m1 + m2 + m3 + m4 + m5) + (dth3*(m4*((l4*sin(th1 + th2 + th3 + th4))/2 + l3*sin(th1 + th2 + th3)) + (l3*m3*sin(th1 + th2 + th3))/2))/(m1 + m2 + m3 + m4 + m5) + (dth4*l4*m4*sin(th1 + th2 + th3 + th4))/(2*(m1 + m2 + m3 + m4 + m5))) - dth1*((dth3*(m4*((l4*sin(th1 + th2 + th3 + th4))/2 + l3*sin(th1 + th2 + th3)) + (l3*m3*sin(th1 + th2 + th3))/2))/(m1 + m2 + m3 + m4 + m5) + (dth1*(m3*(l2*sin(th1 + th2) + l1*sin(th1) + (l3*sin(th1 + th2 + th3))/2) + m5*(l2*sin(th1 + th2) + l1*sin(th1) + (l5*sin(th1 + th2 + th5))/2) + m2*((l2*sin(th1 + th2))/2 + l1*sin(th1)) + m4*((l4*sin(th1 + th2 + th3 + th4))/2 + l2*sin(th1 + th2) + l1*sin(th1) + l3*sin(th1 + th2 + th3)) + (l1*m1*sin(th1))/2))/(m1 + m2 + m3 + m4 + m5) + (dth2*(m4*((l4*sin(th1 + th2 + th3 + th4))/2 + l2*sin(th1 + th2) + l3*sin(th1 + th2 + th3)) + m3*(l2*sin(th1 + th2) + (l3*sin(th1 + th2 + th3))/2) + m5*(l2*sin(th1 + th2) + (l5*sin(th1 + th2 + th5))/2) + (l2*m2*sin(th1 + th2))/2))/(m1 + m2 + m3 + m4 + m5) + (dth4*l4*m4*sin(th1 + th2 + th3 + th4))/(2*(m1 + m2 + m3 + m4 + m5)) + (dth5*l5*m5*sin(th1 + th2 + th5))/(2*(m1 + m2 + m3 + m4 + m5))) - dth4*((dth1*l4*m4*sin(th1 + th2 + th3 + th4))/(2*(m1 + m2 + m3 + m4 + m5)) + (dth2*l4*m4*sin(th1 + th2 + th3 + th4))/(2*(m1 + m2 + m3 + m4 + m5)) + (dth3*l4*m4*sin(th1 + th2 + th3 + th4))/(2*(m1 + m2 + m3 + m4 + m5)) + (dth4*l4*m4*sin(th1 + th2 + th3 + th4))/(2*(m1 + m2 + m3 + m4 + m5))) - dth2*((dth3*(m4*((l4*sin(th1 + th2 + th3 + th4))/2 + l3*sin(th1 + th2 + th3)) + (l3*m3*sin(th1 + th2 + th3))/2))/(m1 + m2 + m3 + m4 + m5) + (dth1*(m4*((l4*sin(th1 + th2 + th3 + th4))/2 + l2*sin(th1 + th2) + l3*sin(th1 + th2 + th3)) + m3*(l2*sin(th1 + th2) + (l3*sin(th1 + th2 + th3))/2) + m5*(l2*sin(th1 + th2) + (l5*sin(th1 + th2 + th5))/2) + (l2*m2*sin(th1 + th2))/2))/(m1 + m2 + m3 + m4 + m5) + (dth2*(m4*((l4*sin(th1 + th2 + th3 + th4))/2 + l2*sin(th1 + th2) + l3*sin(th1 + th2 + th3)) + m3*(l2*sin(th1 + th2) + (l3*sin(th1 + th2 + th3))/2) + m5*(l2*sin(th1 + th2) + (l5*sin(th1 + th2 + th5))/2) + (l2*m2*sin(th1 + th2))/2))/(m1 + m2 + m3 + m4 + m5) + (dth4*l4*m4*sin(th1 + th2 + th3 + th4))/(2*(m1 + m2 + m3 + m4 + m5)) + (dth5*l5*m5*sin(th1 + th2 + th5))/(2*(m1 + m2 + m3 + m4 + m5))) - dth5*((dth1*l5*m5*sin(th1 + th2 + th5))/(2*(m1 + m2 + m3 + m4 + m5)) + (dth2*l5*m5*sin(th1 + th2 + th5))/(2*(m1 + m2 + m3 + m4 + m5)) + (dth5*l5*m5*sin(th1 + th2 + th5))/(2*(m1 + m2 + m3 + m4 + m5))) + (ddth3*(m4*((l4*cos(th1 + th2 + th3 + th4))/2 + l3*cos(th1 + th2 + th3)) + (l3*m3*cos(th1 + th2 + th3))/2))/(m1 + m2 + m3 + m4 + m5) + (ddth2*(m3*(l2*cos(th1 + th2) + (l3*cos(th1 + th2 + th3))/2) + m5*(l2*cos(th1 + th2) + (l5*cos(th1 + th2 + th5))/2) + m4*((l4*cos(th1 + th2 + th3 + th4))/2 + l2*cos(th1 + th2) + l3*cos(th1 + th2 + th3)) + (l2*m2*cos(th1 + th2))/2))/(m1 + m2 + m3 + m4 + m5) + (ddth4*l4*m4*cos(th1 + th2 + th3 + th4))/(2*(m1 + m2 + m3 + m4 + m5)) + (ddth5*l5*m5*cos(th1 + th2 + th5))/(2*(m1 + m2 + m3 + m4 + m5));
% 
% CoM_acc = [xG; zG; dxG; dzG; ddxG; ddzG];

%%
dX = [dq; ddq];

end
